simulink library "SEMACE3_INSTRUMENTATION"  (R2021b)
settings: Solver=VariableStepAuto  StartTime=0.0  StopTime=10.0  RelTol=1e-3
settings Model: Creator=ACH  LastModifiedBy=ACH

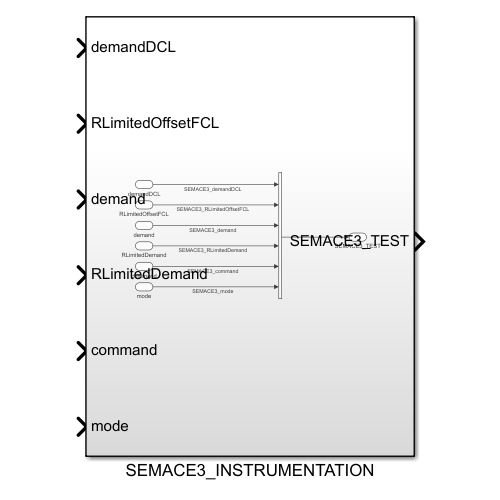
[thumbnail: Simulink's stored preview of the top-level diagram]
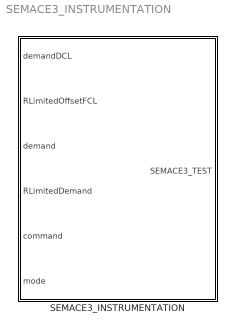
== system SEMACE3_INSTRUMENTATION ==
  SEMACE3_INSTRUMENTATION : Subsystem

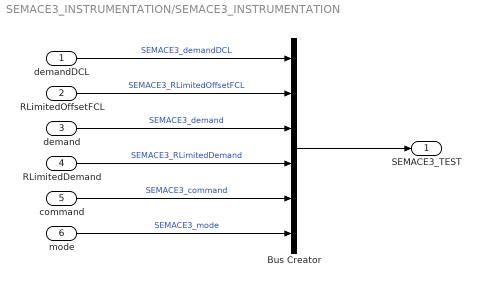
== system SEMACE3_INSTRUMENTATION/SEMACE3_INSTRUMENTATION ==
  demandDCL : Inport
  RLimitedOffsetFCL : Inport  Port=2
  demand : Inport  Port=3
  RLimitedDemand : Inport  Port=4
  command : Inport  Port=5
  mode : Inport  Port=6
  Bus Creator : BusCreator  Inputs=6  OutDataTypeStr=Bus: SEMACE3_TEST
  SEMACE3_TEST : Outport  OutDataTypeStr=Bus: SEMACE3_TEST
  wires:
  mode/1 -> Bus Creator/6  "SEMACE3_mode"
  demand/1 -> Bus Creator/3  "SEMACE3_demand"
  Bus Creator/1 -> SEMACE3_TEST/1
  command/1 -> Bus Creator/5  "SEMACE3_command"
  demandDCL/1 -> Bus Creator/1  "SEMACE3_demandDCL"
  RLimitedOffsetFCL/1 -> Bus Creator/2  "SEMACE3_RLimitedOffsetFCL"
  RLimitedDemand/1 -> Bus Creator/4  "SEMACE3_RLimitedDemand"
